simulink model "lab1"  (R2019b)
settings: Solver=VariableStepAuto  StartTime=0.0  StopTime=1  RelTol=1e-3
undefined symbols (not defined in the file): magnitude
libraries: dspsrcs4 x1, simulink_extras x1
settings Model: Creator=km41417  LastModifiedBy=km41417

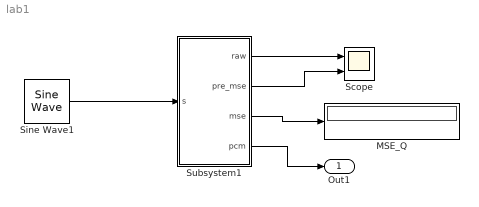
== system lab1 ==
  MSE_Q : Display
  Scope : Scope  NumInputPorts=2
  Sine Wave1 : dspsrcs4/Sine Wave  Amplitude=1  Frequency=1  Phase=0  SampleMode=Continuous  OutComplex=Real  CompMethod=Trigonometric fcn  TableSize=Speed  SampleTime=1/1000  SamplesPerFrame=1  ResetState=Restart at time zero  OutputFrames=off  dataType=double  wordLen=16  udDataType=sfix(16)  fracBitsMode=Best precision  numFracBits=15  OutDataTypeStr=double  LastOutDataTypeStr=double
  Subsystem1 : Subsystem  mask{qint=1/30, qres=8, mseint=1/2048}
      mask prompts: qint "Quantization interval"; qres "Quantization resolution"; mseint "MSE interval"
  Out1 : Outport
  wires:
  Sine Wave1/1 -> Subsystem1/1(s)
  Subsystem1/1(raw) -> Scope/1
  Subsystem1/2(pre_mse) -> Scope/2
  Subsystem1/3(mse) -> MSE_Q/1
  Subsystem1/4("pcm ") -> Out1/1

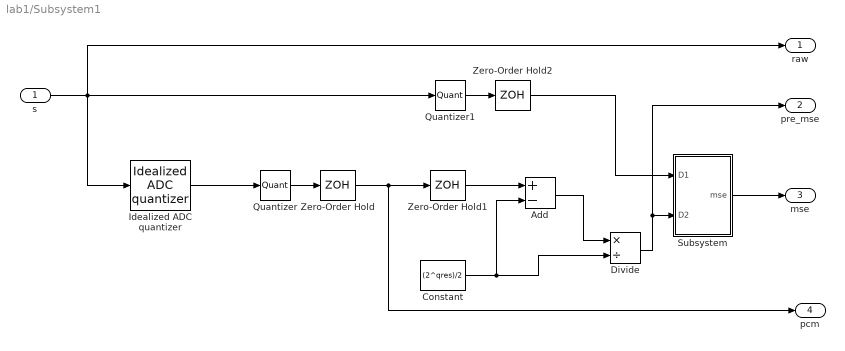
== system lab1/Subsystem1 ==
  s : Inport
  Add : Sum  Inputs=+-
  Constant : Constant  Value=(2^qres)/2
  Divide : Product  Inputs=*/
  Idealized ADC quantizer : simulink_extras/Additional Discrete/Idealized ADC quantizer  NumberOfConverterBits=qres  Vmin=-1  Vmax=1  OutputDataType=double  OutputNegativeValues=off
      settings: SourceProductName=Simulink
  Quantizer : Quantizer  QuantizationInterval=qint
  Quantizer1 : Quantizer  QuantizationInterval=mseint
  Subsystem : Subsystem
  Zero-Order Hold : ZeroOrderHold  SampleTime=qint
  Zero-Order Hold1 : ZeroOrderHold  SampleTime=mseint
  Zero-Order Hold2 : ZeroOrderHold  SampleTime=mseint
  raw : Outport
  pre_mse : Outport  Port=2
  mse : Outport  Port=3
  "pcm " : Outport  Port=4
  wires:
  s/1 -> raw/1, Idealized ADC quantizer/1, Quantizer1/1
  Subsystem/1(mse) -> mse/1
  Constant/1 -> Add/2, Divide/2
  Zero-Order Hold/1 -> "pcm "/1, Zero-Order Hold1/1
  Zero-Order Hold1/1 -> Add/1
  Add/1 -> Divide/1
  Divide/1 -> pre_mse/1, Subsystem/2("D2 ")
  Zero-Order Hold2/1 -> Subsystem/1("D1 ")
  Quantizer1/1 -> Zero-Order Hold2/1
  Quantizer/1 -> Zero-Order Hold/1
  Idealized ADC quantizer/1 -> Quantizer/1

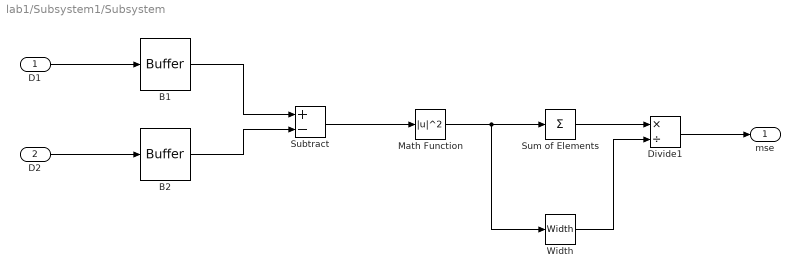
== system lab1/Subsystem1/Subsystem ==
  "D1 " : Inport
  "D2 " : Inport  Port=2
  B1 : Buffer  OutputFrames=off
  "B2 " : Buffer  OutputFrames=off
  Divide1 : Product  Inputs=*/
  Math Function : Math  Operator=magnitude^2  SignedPower=off  SaturateOnIntegerOverflow=on
  Subtract : Sum  Inputs=+-
  Sum of Elements : Sum  Inputs=+
  Width : Width
  mse : Outport
  wires:
  "D2 "/1 -> "B2 "/1
  "B2 "/1 -> Subtract/2
  "D1 "/1 -> B1/1
  Subtract/1 -> Math Function/1
  Math Function/1 -> Width/1, Sum of Elements/1
  B1/1 -> Subtract/1
  Sum of Elements/1 -> Divide1/1
  Divide1/1 -> mse/1
  Width/1 -> Divide1/2
